simulink model "BMP180_SF3"  (R2018a)
settings: Solver=FixedStepDiscrete  StartTime=0.0  StopTime=inf  FixedStep=0.05  RelTol=1e-3  EnableMultiTasking=on
InitFcn:
  | Ts=0.05;
libraries: arduinolib x3
settings Model: EnablePacing=on  ExtModeTrigDuration=2  Creator=Marc  LastModifiedBy=Marc
settings DataIOCC: SaveOutput=off  SaveTime=off  TimeSaveName=time
settings OptimizationCC: LifeSpan=1  MaxStackSize=64
settings DebuggingCC: AllowSymbolicDim=off  SFUnexpectedBacktrackingDiag=warning  SFNoUnconditionalDefaultTransitionDiag=warning  SFExecutionAtInitializationDiag=none
settings HardwareCC: ProdBitPerInt=16  ProdBitPerPointer=16  ProdBitPerSizeT=16  ProdBitPerPtrDiffT=16  ProdLargestAtomicFloat=None  ProdWordSize=8  ProdHWDeviceType=Atmel->AVR  UseEmbeddedCoderFeatures=off  UseSimulinkCoderFeatures=off
settings ModelReferenceCC: PropagateSignalLabelsOutOfModel=off
settings RTWCC: SystemTargetFile=ert.tlc  HardwareBoard=Arduino Mega 2560  TemplateMakefile=ert_default_tmf  Toolchain=Arduino AVR  BuildConfiguration=Faster Runs
settings CodeAppCC: MangleLength=10  StateflowObjectComments=on
settings ERTTargetCC: MultiwordLength=2048  ERTCustomFileBanners=off  SupportContinuousTime=on  SupportNonInlinedSFcns=on  RemoveResetFunc=off  SupportVariableSizeSignals=on  ModelStepFunctionPrototypeControlCompliant=off  ConvertIfToSwitch=off  SuppressUnreachableDefaultCases=off
settings ConfigComp: CovMetricSettings=dw  CovHtmlReporting=on  CovSaveCumulativeToWorkspaceVar=on  CovSaveSingleToWorkspaceVar=on  CovExternalEMLEnable=off
settings SimscapeCC: SimscapeNormalizeSystem=off

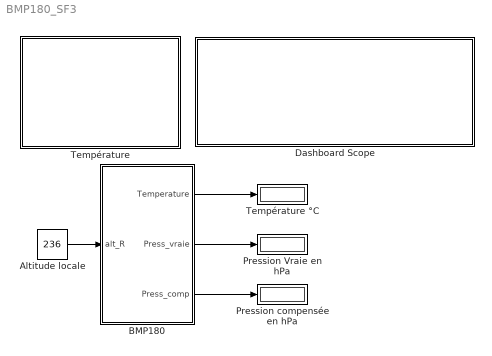
== system BMP180_SF3 ==
  Altitude locale : Constant  Value=236  OutDataTypeStr=single
  BMP180 : Stateflow chart  TreatAsAtomicUnit=on
  Dashboard Scope : Subsystem  DialogController=hmiCreateDDGDialog  IsWebBlock=on  mask(MWDashboardBlock){webBlockId=15e4855c-e0cb-4c4a-bee6-d3d92fed0d0c, webBlockType=sdiscope, ShowInitialText=on, HMISrcModelName=BMP180_SF2}
      mask prompts: webBlockId "WebBlock Id"; webBlockType "WebBlock Type"; HMISrcModelName "Source Model"
      mask help: SimulinkHMI:dialogs:HMIScopeDialogDesc
      mask Help: helpview([docroot '/mapfiles/simulink.map'], 'hmi_scope')
      mask Display:
      | if strcmp(get_param(bdroot(gcb),'BlockDiagramType'), 'library')
      |     image([(matlabroot) '/toolbox/simulink/hmi/icons/DashboardScope.png']);
      | end
  Pression Vraie en hPa : Display
      settings: Format=bank
  Pression compensée en hPa : Display
      settings: Format=bank
  Température : Subsystem  DialogController=hmiCreateDDGDialog  IsWebBlock=on  mask(MWDashboardBlock){webBlockId=f9d7495a-ec57-46ff-b23a-6e99dd3e9f83, webBlockType=semicirculargauge, ShowInLibBrowser=on, ShowInitialText=on, HMISrcModelName=BMP180_SF2}
      mask prompts: webBlockId "WebBlock Id"; webBlockType "WebBlock Type"; HMISrcModelName "Source Model"
      mask help: SimulinkHMI:dialogs:SemicircularGaugeDialogDesc
      mask Help: helpview([docroot '/mapfiles/simulink.map'], 'hmi_half_gauge')
      mask Display:
      | if strcmp(get_param(bdroot(gcb),'BlockDiagramType'), 'library')
      |     image([(matlabroot) '/toolbox/simulink/hmi/icons/SemicircularGauge.png']);
      | end
  Température °C : Display
      settings: Format=bank
  wires:
  BMP180/3(Press_comp) -> Pression compensée en hPa/1
  BMP180/1(Temperature) -> Température °C/1
  Altitude locale/1 -> BMP180/1(alt_R)
  BMP180/2(Press_vraie) -> Pression Vraie en hPa/1

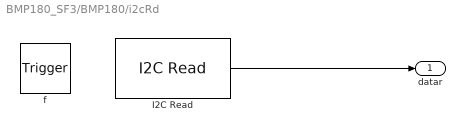
== system BMP180_SF3/BMP180/i2cRd ==
  f : TriggerPort  TriggerType=function-call  VariantControl=Variant  SampleTime=-1
      settings: CopyFcn=Stateflow.SLINSF.SimulinkMan.removeBlockPreDeleteFcn  PreDeleteFcn=Stateflow.SLINSF.SimulinkMan.unsafePredeleteFcn
  I2C Read : arduinolib/I2C Read  SlaveAddress_=hex2dec( '77' )  RegisterAddressEnable=on  RegisterAddress_=hex2dec( 'F6' )  Datatype=uint16  ByteOrder=Big Endian  Datalength_=1  SampleTime_=-1  blockPlatform=arduino
      settings: SourceProductName=Simulink Support Package for Arduino Hardware  SourceProductBaseCode=ARDUINO
  datar : Outport  OutDataTypeStr=uint16  Unit=1  PortDimensions=1
  wires:
  I2C Read/1 -> datar/1

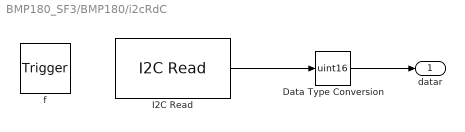
== system BMP180_SF3/BMP180/i2cRdC ==
  f : TriggerPort  TriggerType=function-call  VariantControl=Variant  SampleTime=-1
      settings: CopyFcn=Stateflow.SLINSF.SimulinkMan.removeBlockPreDeleteFcn  PreDeleteFcn=Stateflow.SLINSF.SimulinkMan.unsafePredeleteFcn
  Data Type Conversion : DataTypeConversion  OutDataTypeStr=uint16
  I2C Read : arduinolib/I2C Read  SlaveAddress_=hex2dec( '77' )  RegisterAddressEnable=on  RegisterAddress_=hex2dec( 'AA' )  Datatype=uint16  ByteOrder=Big Endian  Datalength_=11  SampleTime_=-1  blockPlatform=arduino
      settings: SourceProductName=Simulink Support Package for Arduino Hardware  SourceProductBaseCode=ARDUINO
  datar : Outport  OutDataTypeStr=uint16  Unit=1  PortDimensions=11
  wires:
  I2C Read/1 -> Data Type Conversion/1
  Data Type Conversion/1 -> datar/1

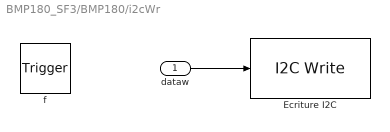
== system BMP180_SF3/BMP180/i2cWr ==
  dataw : Inport  OutDataTypeStr=uint16  Unit=1  PortDimensions=1
  f : TriggerPort  TriggerType=function-call  VariantControl=Variant  SampleTime=-1
      settings: CopyFcn=Stateflow.SLINSF.SimulinkMan.removeBlockPreDeleteFcn  PreDeleteFcn=Stateflow.SLINSF.SimulinkMan.unsafePredeleteFcn
  Ecriture I2C : arduinolib/I2C Write  Priority=1  SlaveAddress_=hex2dec( '77' )  RegisterAddressEnable=off  RegisterAddress_=hex2dec( '6B' )  Datatype=uint16  ByteOrder=Big Endian  blockPlatform=arduino
      settings: SourceProductName=Simulink Support Package for Arduino Hardware  SourceProductBaseCode=ARDUINO
  wires:
  dataw/1 -> Ecriture I2C/1

== system BMP180_SF3/Dashboard Scope ==

== system BMP180_SF3/Température ==

== stateflow chart BMP180_SF3/BMP180 ==
  state Lecture_constantes
    entry:
    val=i2cRdC;
    AC1=single(typecast(uint16(val(1:1)), 'int16'));
    AC2=single(typecast(uint16(val(2:2)), 'int16'));
    AC3=single(typecast(uint16(val(3:3)), 'int16'));
    AC4=single(uint16(val(4:4)));
    AC5=single(uint16(val(5:5)));
    AC6=single(uint16(val(6:6)));
    B1=single(typecast(uint16(val(7:7)), 'int16'));
    B2=single(typecast(uint16(val(8:8)), 'int16'));
    MB=single(typecast(uint16(val(9:9)), 'int16'));
    MC=single(typecast(uint16(val(10:10)), 'int16'));
    MD=single(typecast(uint16(val(11:11)), 'int16'));
    %lecture des constance et conversion en simple précision
  note: 25ms mini entre conversion et lecture
      | Ts = 50ms donc OK
  state Debut_conversion
    entry:
    i2cWr(uint16(hex2dec( 'F42E' )));%start conversion
  state Lecture_donnees_temperature
    entry:
    UT=single(i2cRd);%valeur brut de la temperature
    X1=(UT-AC6)*AC5/2^15;
    X2=MC*2^11/(X1+MD);
    B5=X1+X2;
    Temperature=((B5+8)/2^4)/10;
  state Debut_conversion1
    entry:
    i2cWr(uint16(hex2dec( 'F434' )));%start conv. OSS=0    4ms
  state Lecture_donnees_Pression
    entry:
    UP=single(i2cRd);%pression non compensée
    B6=B5-4000;
    X1=(B2*(B6*(B6/2^12))/2^11);
    X2=AC2*B6/2^11;
    X3=X1+X2;
    B3=((AC1*4+X3)+2)/4;
    X1=AC3*B6/2^13;
    X2=(B1*(B6*B6/2^12))/2^16;
    X3=((X1+X2)+2)/4;
    B4=AC4*(X3+32768)/2^15;
    B7=(UP-B3)*50000;
    if B7 <8*16^8
    p=(B7*2/B4);
    else
    p=(B7/B4)*2;
    end
    X1=(p/2^8)^2;
    X1=(X1*3038)/2^16;
    X2=(-7357*p)/2^16;
    Press_vraie= (p+(X1+X2+3791)/2^4)/100;
    Press_comp=Press_vraie/((1-alt_R/44330)^5.255);
  state datar = i2cRdC [function]
  state datar = i2cRd [function]
  state i2cWr(dataw) [function]
  (default) -> Lecture_constantes
  Lecture_constantes -> Debut_conversion
  Lecture_donnees_Pression -> Debut_conversion : after(1,sec)
  Debut_conversion -> Lecture_donnees_temperature
  Lecture_donnees_temperature -> Debut_conversion1
  Debut_conversion1 -> Lecture_donnees_Pression
  data: datar function_output uint16 size=11; datar function_output uint16 size=1; dataw function_input uint16 size=1; Temperature output single size=1; val local uint16 size=11; AC1 local single size=1; AC2 local single size=1; AC3 local single size=1; AC4 local single size=1; B1 local single size=1; B2 local single size=1; MB local single size=1; X2 local single size=1; B5 local single size=1; AC5 local single size=1; AC6 local single size=1; MC local single size=1; MD local single size=1; UT local single size=1; X1 local single size=1; UP local single size=1; B3 local single size=1; B4 local single size=1; B7 local single size=1; X3 local single size=1; B6 local single size=1; alt_R input single size=1; Press_vraie output single size=1; Press_comp output single size=1; p local single size=1
